simulink model "M10B39_V2"  (R2025a)
settings: Solver=ode23tb  StartTime=0.0  StopTime=1000  FixedStep=0.001  RelTol=1e-3  EnableMultiTasking=on
InitFcn:
  | clear;
  | initAll_V2;
  | %set_param('M10B39/Python2Sim','value','zeros(1,16)');
values from neighbouring files (symbols this model uses):
  acom = 100    [initAll.m]    (also in initAll_V2.m)
  bcom = 50    [initAll.m]    (also in initAll_V2.m)
  commun = 0*commun    [initAll.m]    (also in initAll_V2.m)
  DataDelay = 0.0*DataDelay    [initAll.m]    (also in initAll_V2.m)
  fB = 50    [initAll.m]    (also in initAll_V2.m)
  Geninit = Generator_init(opdata,SynMach_in_gidx)    [initAll.m]    (also in initAll_V2.m)
  lam = 100    [initAll.m]    (also in initAll_V2.m)
  loadnode = 31    [initAll_V2.m]
  loadsize = 16.2714    [initAll_V2.m]
  SgridB = 100    [initAll.m]    (also in initAll_V2.m)
  wB = 2*pi*fB    (= 314.159265359)    [initAll.m]    (also in initAll_V2.m)
undefined symbols (not defined in the file or in its folder): AVm0, c1, c2, c3, c4, c5, c6, cp_nom, ESinit, lambda_nom, P_wind_base, Pelec_base, Pnom, Windinit, YY_load
libraries: spsBistableLib x13, simulink_extras x5, powerlib_meascontrol x2, simulink x1
(part 2 of 11)

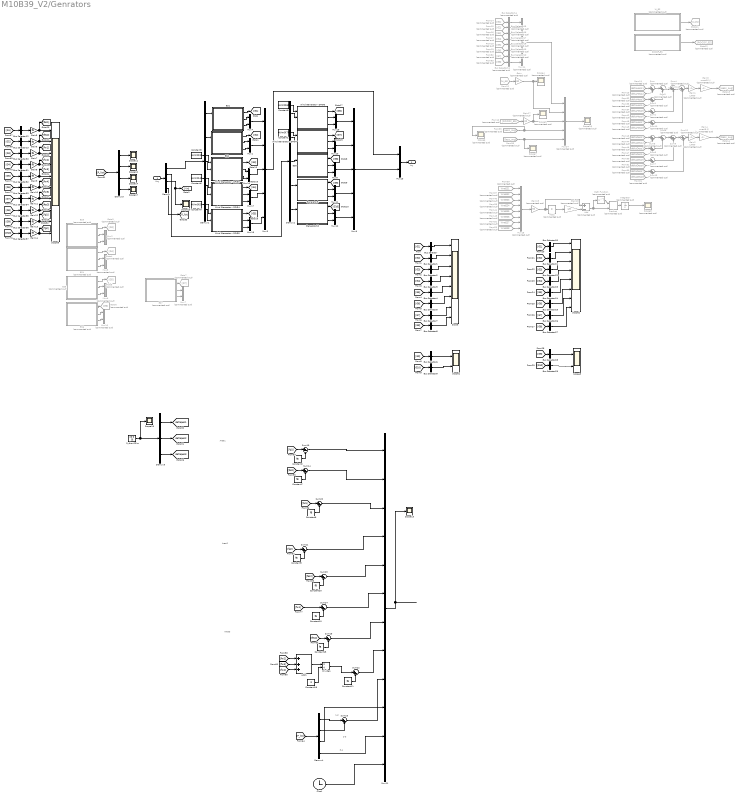
== system M10B39_V2/Genrators ==
  note: 3-1
  note: Area3
  note: 1-2
  note: 2-3
  note: Area2
  note: Area1
  Vxy : Inport
  Add : Sum  Commented=on  Inputs=+-
  Add1 : Sum  Inputs=+++
  Add2 : Sum  Commented=on  Inputs=+
  Bus Selector{,1..5,7..8,12..13,30..35} (16 alike) : BusSelector  OutputSignals=w
  Bus Selector{10..11,14..19} (8 alike) : BusSelector  Commented=on  OutputSignals=Pe
  Bus Selector{20..29} (10 alike) : BusSelector  OutputSignals=Pe
  Bus Selector{6,9,36..37} (4 alike) : BusSelector  OutputSignals=f
  Clock : Clock
  Constant1 : Constant  Value=AVm0(7)
  Constant{2,7..11,15,20} (8 alike) : Constant  Value=fB
  Constant18 : Constant  Value=3
  Constant3 : Constant  Value=AVm0(3)
  Constant4 : Constant  Value=AVm0(5)
  Constant5 : Constant  Value=AVm0(6)
  Constant6 : Constant  Value=AVm0(4)
  Demux : Demux  Outputs=[10 10 29 4]
      settings: DisplayOption=none
  Demux1 : Demux  Outputs=5
      settings: DisplayOption=none
  Demux2 : Demux  Outputs=5
      settings: DisplayOption=none
  Demux3 : Demux
  Demux4 : Demux
  Demux5 : Demux  Outputs=3
  Divide1 : Product  Inputs=*/
  ES1 : Subsystem  mask{SvscB=ESinit.SvscBi(1), SgridB=SgridB, Kppll_VSC=ESinit.Kppll(1), Kipll_VSC=ESinit.Kipll(1), Dels_hvdc=ESinit.Dels_hvdc(1), Lpr=ESinit.Lpr(1), Rpr=ESinit.Rpr(1), wB=wB, Is_xA_0=ESinit.Isx0(1), Is_yA_0=ESinit.Isy0(1), KpP_VSC_A=ESinit.KpP(1), KiP_VSC_A=ESinit.KiP(1), KpId_VSC_A=ESinit.KpId(1), KiId_VSC_A=ESinit.KiId(1), KpQ_VSC_A=ESinit.KpQ(1), KiQ_VSC_A=ESinit.KiQ(1), KpIq_VSC_A=ESinit.KpIq(1), KiIq_VSC_A=ESinit.KiIq(1), Md_A_0=ESinit.Md0(1), Mq_A_0=ESinit.Mq0(1), Nd_A_0=ESinit.Nd0(1), Nq_A_0=ESinit.Nq0(1), KIR=ESinit.Kir(1), Kdroop=ESinit.Kdroop(1), Kdistributed=ESinit.Kdistributed(1), Kdistributed_d=ESinit.Kdistributed_d(1), Kpac_VSC_A=ESinit.Kpac(1), Kiac_VSC_A=ESinit.Kiac(1), P0=ESinit.P0(1), Q0=ESinit.Q0(1), usd0=ESinit.Usd0(1)}
      mask prompts: Kppll_VSC "Kppll"; Kipll_VSC "Kipll"; KpP_VSC_A "KpP"; KiP_VSC_A "KiP"; KpId_VSC_A "KpId"; KiId_VSC_A "KiId"; KpQ_VSC_A "KpQ"; KiQ_VSC_A "KiQ"; KpIq_VSC_A "KpIq"; KiIq_VSC_A "KiIq"; Kpac_VSC_A "Kpac"; Kiac_VSC_A "Kiac"
      mask DialogControl Container48 Prompt: Base value
      mask DialogControl Container7 Prompt: PLL
      mask DialogControl Container5 Prompt: Control parameter
      mask DialogControl Container8 Prompt: inital value
      mask DialogControl Container9 Prompt: AC side
      mask DialogControl Container10 Prompt: Parameter
      mask DialogControl Container11 Prompt: Initial value
      mask DialogControl Container18 Prompt: Control parameter
      mask DialogControl Container19 Prompt: d_axis_control parameter
      mask DialogControl Container23 Prompt: d_axis_control=1
      mask DialogControl Container26 Prompt: inner current control
      mask DialogControl Container21 Prompt: q_axis_control parameter
      mask DialogControl Container29 Prompt: q_axis_control=1
      mask DialogControl Container31 Prompt: inner current control
      mask DialogControl Container22 Prompt: inital value
      mask DialogControl Container35 Prompt: outer controller
      mask DialogControl Container36 Prompt: inner control
      mask DialogControl Container27 Prompt: Inertia control
      mask DialogControl Container28 Prompt: droop control
      mask DialogControl Container300 Prompt: distributed control
      mask DialogControl Container301 Prompt: Droop distributed control
      mask DialogControl Container40 Prompt: usdq_control
      mask DialogControl Container41 Prompt: PQinitial
      mask DialogControl Container42 Prompt: usd0initial
  ES2 : Subsystem  mask{SvscB=ESinit.SvscBi(2), SgridB=SgridB, Kppll_VSC=ESinit.Kppll(2), Kipll_VSC=ESinit.Kipll(2), Dels_hvdc=ESinit.Dels_hvdc(2), Lpr=ESinit.Lpr(2), Rpr=ESinit.Rpr(2), wB=wB, Is_xA_0=ESinit.Isx0(2), Is_yA_0=ESinit.Isy0(2), KpP_VSC_A=ESinit.KpP(2), KiP_VSC_A=ESinit.KiP(2), KpId_VSC_A=ESinit.KpId(2), KiId_VSC_A=ESinit.KiId(2), KpQ_VSC_A=ESinit.KpQ(2), KiQ_VSC_A=ESinit.KiQ(2), KpIq_VSC_A=ESinit.KpIq(2), KiIq_VSC_A=ESinit.KiIq(2), Md_A_0=ESinit.Md0(2), Mq_A_0=ESinit.Mq0(2), Nd_A_0=ESinit.Nd0(2), Nq_A_0=ESinit.Nq0(2), KIR=ESinit.Kir(2), Kdroop=ESinit.Kdroop(2), Kdistributed=ESinit.Kdistributed(2), Kdistributed_d=ESinit.Kdistributed_d(2), Kpac_VSC_A=ESinit.Kpac(2), Kiac_VSC_A=ESinit.Kiac(2), P0=ESinit.P0(2), Q0=ESinit.Q0(2), usd0=ESinit.Usd0(2)}
      mask prompts: Kppll_VSC "Kppll"; Kipll_VSC "Kipll"; KpP_VSC_A "KpP"; KiP_VSC_A "KiP"; KpId_VSC_A "KpId"; KiId_VSC_A "KiId"; KpQ_VSC_A "KpQ"; KiQ_VSC_A "KiQ"; KpIq_VSC_A "KpIq"; KiIq_VSC_A "KiIq"; Kpac_VSC_A "Kpac"; Kiac_VSC_A "Kiac"
      mask DialogControl Container48 Prompt: Base value
      mask DialogControl Container7 Prompt: PLL
      mask DialogControl Container5 Prompt: Control parameter
      mask DialogControl Container8 Prompt: inital value
      mask DialogControl Container9 Prompt: AC side
      mask DialogControl Container10 Prompt: Parameter
      mask DialogControl Container11 Prompt: Initial value
      mask DialogControl Container18 Prompt: Control parameter
      mask DialogControl Container19 Prompt: d_axis_control parameter
      mask DialogControl Container23 Prompt: d_axis_control=1
      mask DialogControl Container26 Prompt: inner current control
      mask DialogControl Container21 Prompt: q_axis_control parameter
      mask DialogControl Container29 Prompt: q_axis_control=1
      mask DialogControl Container31 Prompt: inner current control
      mask DialogControl Container22 Prompt: inital value
      mask DialogControl Container35 Prompt: outer controller
      mask DialogControl Container36 Prompt: inner control
      mask DialogControl Container27 Prompt: Inertia control
      mask DialogControl Container28 Prompt: droop control
      mask DialogControl Container300 Prompt: distributed control
      mask DialogControl Container301 Prompt: Droop distributed control
      mask DialogControl Container40 Prompt: usdq_control
      mask DialogControl Container41 Prompt: PQinitial
      mask DialogControl Container42 Prompt: usd0initial
  ES3 : Subsystem  Commented=on  mask{SvscB=ESinit.SvscBi(3), SgridB=SgridB, Kppll_VSC=ESinit.Kppll(3), Kipll_VSC=ESinit.Kipll(3), Dels_hvdc=ESinit.Dels_hvdc(3), Lpr=ESinit.Lpr(3), Rpr=ESinit.Rpr(3), wB=wB, Is_xA_0=ESinit.Isx0(3), Is_yA_0=ESinit.Isy0(3), KpP_VSC_A=ESinit.KpP(3), KiP_VSC_A=ESinit.KiP(3), KpId_VSC_A=ESinit.KpId(3), KiId_VSC_A=ESinit.KiId(3), KpQ_VSC_A=ESinit.KpQ(3), KiQ_VSC_A=ESinit.KiQ(3), KpIq_VSC_A=ESinit.KpIq(3), KiIq_VSC_A=ESinit.KiIq(3), Md_A_0=ESinit.Md0(3), Mq_A_0=ESinit.Mq0(3), Nd_A_0=ESinit.Nd0(3), Nq_A_0=ESinit.Nq0(3), KIR=ESinit.Kir(3), Kdroop=ESinit.Kdroop(3), Kdistributed=ESinit.Kdistributed(3), Kdistributed_d=ESinit.Kdistributed_d(3), Kpac_VSC_A=ESinit.Kpac(3), Kiac_VSC_A=ESinit.Kiac(3), P0=ESinit.P0(3), Q0=ESinit.Q0(3), usd0=ESinit.Usd0(3)}
      mask prompts: Kppll_VSC "Kppll"; Kipll_VSC "Kipll"; KpP_VSC_A "KpP"; KiP_VSC_A "KiP"; KpId_VSC_A "KpId"; KiId_VSC_A "KiId"; KpQ_VSC_A "KpQ"; KiQ_VSC_A "KiQ"; KpIq_VSC_A "KpIq"; KiIq_VSC_A "KiIq"; Kpac_VSC_A "Kpac"; Kiac_VSC_A "Kiac"
      mask DialogControl Container48 Prompt: Base value
      mask DialogControl Container7 Prompt: PLL
      mask DialogControl Container5 Prompt: Control parameter
      mask DialogControl Container8 Prompt: inital value
      mask DialogControl Container9 Prompt: AC side
      mask DialogControl Container10 Prompt: Parameter
      mask DialogControl Container11 Prompt: Initial value
      mask DialogControl Container18 Prompt: Control parameter
      mask DialogControl Container19 Prompt: d_axis_control parameter
      mask DialogControl Container23 Prompt: d_axis_control=1
      mask DialogControl Container26 Prompt: inner current control
      mask DialogControl Container21 Prompt: q_axis_control parameter
      mask DialogControl Container29 Prompt: q_axis_control=1
      mask DialogControl Container31 Prompt: inner current control
      mask DialogControl Container22 Prompt: inital value
      mask DialogControl Container35 Prompt: outer controller
      mask DialogControl Container36 Prompt: inner control
      mask DialogControl Container27 Prompt: Inertia control
      mask DialogControl Container28 Prompt: droop control
      mask DialogControl Container300 Prompt: distributed control
      mask DialogControl Container301 Prompt: Droop distributed control
      mask DialogControl Container40 Prompt: usdq_control
      mask DialogControl Container41 Prompt: PQinitial
      mask DialogControl Container42 Prompt: usd0initial
  ES4 : Subsystem  Commented=on  mask{SvscB=ESinit.SvscBi(4), SgridB=SgridB, Kppll_VSC=ESinit.Kppll(4), Kipll_VSC=ESinit.Kipll(4), Dels_hvdc=ESinit.Dels_hvdc(4), Lpr=ESinit.Lpr(4), Rpr=ESinit.Rpr(4), wB=wB, Is_xA_0=ESinit.Isx0(4), Is_yA_0=ESinit.Isy0(4), KpP_VSC_A=ESinit.KpP(4), KiP_VSC_A=ESinit.KiP(4), KpId_VSC_A=ESinit.KpId(4), KiId_VSC_A=ESinit.KiId(4), KpQ_VSC_A=ESinit.KpQ(4), KiQ_VSC_A=ESinit.KiQ(4), KpIq_VSC_A=ESinit.KpIq(4), KiIq_VSC_A=ESinit.KiIq(4), Md_A_0=ESinit.Md0(4), Mq_A_0=ESinit.Mq0(4), Nd_A_0=ESinit.Nd0(4), Nq_A_0=ESinit.Nq0(4), KIR=ESinit.Kir(4), Kdroop=ESinit.Kdroop(4), Kdistributed=ESinit.Kdistributed(4), Kdistributed_d=ESinit.Kdistributed_d(4), Kpac_VSC_A=ESinit.Kpac(4), Kiac_VSC_A=ESinit.Kiac(4), P0=ESinit.P0(4), Q0=ESinit.Q0(4), usd0=ESinit.Usd0(4)}
      mask prompts: Kppll_VSC "Kppll"; Kipll_VSC "Kipll"; KpP_VSC_A "KpP"; KiP_VSC_A "KiP"; KpId_VSC_A "KpId"; KiId_VSC_A "KiId"; KpQ_VSC_A "KpQ"; KiQ_VSC_A "KiQ"; KpIq_VSC_A "KpIq"; KiIq_VSC_A "KiIq"; Kpac_VSC_A "Kpac"; Kiac_VSC_A "Kiac"
      mask DialogControl Container48 Prompt: Base value
      mask DialogControl Container7 Prompt: PLL
      mask DialogControl Container5 Prompt: Control parameter
      mask DialogControl Container8 Prompt: inital value
      mask DialogControl Container9 Prompt: AC side
      mask DialogControl Container10 Prompt: Parameter
      mask DialogControl Container11 Prompt: Initial value
      mask DialogControl Container18 Prompt: Control parameter
      mask DialogControl Container19 Prompt: d_axis_control parameter
      mask DialogControl Container23 Prompt: d_axis_control=1
      mask DialogControl Container26 Prompt: inner current control
      mask DialogControl Container21 Prompt: q_axis_control parameter
      mask DialogControl Container29 Prompt: q_axis_control=1
      mask DialogControl Container31 Prompt: inner current control
      mask DialogControl Container22 Prompt: inital value
      mask DialogControl Container35 Prompt: outer controller
      mask DialogControl Container36 Prompt: inner control
      mask DialogControl Container27 Prompt: Inertia control
      mask DialogControl Container28 Prompt: droop control
      mask DialogControl Container300 Prompt: distributed control
      mask DialogControl Container301 Prompt: Droop distributed control
      mask DialogControl Container40 Prompt: usdq_control
      mask DialogControl Container41 Prompt: PQinitial
      mask DialogControl Container42 Prompt: usd0initial
  ES5 : Subsystem  Commented=on  mask{SvscB=ESinit.SvscBi(5), SgridB=SgridB, Kppll_VSC=ESinit.Kppll(5), Kipll_VSC=ESinit.Kipll(5), Dels_hvdc=ESinit.Dels_hvdc(5), Lpr=ESinit.Lpr(5), Rpr=ESinit.Rpr(5), wB=wB, Is_xA_0=ESinit.Isx0(5), Is_yA_0=ESinit.Isy0(5), KpP_VSC_A=ESinit.KpP(5), KiP_VSC_A=ESinit.KiP(5), KpId_VSC_A=ESinit.KpId(5), KiId_VSC_A=ESinit.KiId(5), KpQ_VSC_A=ESinit.KpQ(5), KiQ_VSC_A=ESinit.KiQ(5), KpIq_VSC_A=ESinit.KpIq(5), KiIq_VSC_A=ESinit.KiIq(5), Md_A_0=ESinit.Md0(5), Mq_A_0=ESinit.Mq0(5), Nd_A_0=ESinit.Nd0(5), Nq_A_0=ESinit.Nq0(5), KIR=ESinit.Kir(5), Kdroop=ESinit.Kdroop(5), Kdistributed=ESinit.Kdistributed(5), Kdistributed_d=ESinit.Kdistributed_d(5), Kpac_VSC_A=ESinit.Kpac(5), Kiac_VSC_A=ESinit.Kiac(5), P0=ESinit.P0(5), Q0=ESinit.Q0(5), usd0=ESinit.Usd0(5)}
      mask prompts: Kppll_VSC "Kppll"; Kipll_VSC "Kipll"; KpP_VSC_A "KpP"; KiP_VSC_A "KiP"; KpId_VSC_A "KpId"; KiId_VSC_A "KiId"; KpQ_VSC_A "KpQ"; KiQ_VSC_A "KiQ"; KpIq_VSC_A "KpIq"; KiIq_VSC_A "KiIq"; Kpac_VSC_A "Kpac"; Kiac_VSC_A "Kiac"
      mask DialogControl Container48 Prompt: Base value
      mask DialogControl Container7 Prompt: PLL
      mask DialogControl Container5 Prompt: Control parameter
      mask DialogControl Container8 Prompt: inital value
      mask DialogControl Container9 Prompt: AC side
      mask DialogControl Container10 Prompt: Parameter
      mask DialogControl Container11 Prompt: Initial value
      mask DialogControl Container18 Prompt: Control parameter
      mask DialogControl Container19 Prompt: d_axis_control parameter
      mask DialogControl Container23 Prompt: d_axis_control=1
      mask DialogControl Container26 Prompt: inner current control
      mask DialogControl Container21 Prompt: q_axis_control parameter
      mask DialogControl Container29 Prompt: q_axis_control=1
      mask DialogControl Container31 Prompt: inner current control
      mask DialogControl Container22 Prompt: inital value
      mask DialogControl Container35 Prompt: outer controller
      mask DialogControl Container36 Prompt: inner control
      mask DialogControl Container27 Prompt: Inertia control
      mask DialogControl Container28 Prompt: droop control
      mask DialogControl Container300 Prompt: distributed control
      mask DialogControl Container301 Prompt: Droop distributed control
      mask DialogControl Container40 Prompt: usdq_control
      mask DialogControl Container41 Prompt: PQinitial
      mask DialogControl Container42 Prompt: usd0initial
  ES6 : Subsystem  Commented=on  mask{SvscB=ESinit.SvscBi(6), SgridB=SgridB, Kppll_VSC=ESinit.Kppll(6), Kipll_VSC=ESinit.Kipll(6), Dels_hvdc=ESinit.Dels_hvdc(6), Lpr=ESinit.Lpr(6), Rpr=ESinit.Rpr(6), wB=wB, Is_xA_0=ESinit.Isx0(6), Is_yA_0=ESinit.Isy0(6), KpP_VSC_A=ESinit.KpP(6), KiP_VSC_A=ESinit.KiP(6), KpId_VSC_A=ESinit.KpId(6), KiId_VSC_A=ESinit.KiId(6), KpQ_VSC_A=ESinit.KpQ(6), KiQ_VSC_A=ESinit.KiQ(6), KpIq_VSC_A=ESinit.KpIq(6), KiIq_VSC_A=ESinit.KiIq(6), Md_A_0=ESinit.Md0(6), Mq_A_0=ESinit.Mq0(6), Nd_A_0=ESinit.Nd0(6), Nq_A_0=ESinit.Nq0(6), KIR=ESinit.Kir(6), Kdroop=ESinit.Kdroop(6), Kdistributed=ESinit.Kdistributed(6), Kdistributed_d=ESinit.Kdistributed_d(6), Kpac_VSC_A=ESinit.Kpac(6), Kiac_VSC_A=ESinit.Kiac(6), P0=ESinit.P0(6), Q0=ESinit.Q0(6), usd0=ESinit.Usd0(6)}
      mask prompts: Kppll_VSC "Kppll"; Kipll_VSC "Kipll"; KpP_VSC_A "KpP"; KiP_VSC_A "KiP"; KpId_VSC_A "KpId"; KiId_VSC_A "KiId"; KpQ_VSC_A "KpQ"; KiQ_VSC_A "KiQ"; KpIq_VSC_A "KpIq"; KiIq_VSC_A "KiIq"; Kpac_VSC_A "Kpac"; Kiac_VSC_A "Kiac"
      mask DialogControl Container48 Prompt: Base value
      mask DialogControl Container7 Prompt: PLL
      mask DialogControl Container5 Prompt: Control parameter
      mask DialogControl Container8 Prompt: inital value
      mask DialogControl Container9 Prompt: AC side
      mask DialogControl Container10 Prompt: Parameter
      mask DialogControl Container11 Prompt: Initial value
      mask DialogControl Container18 Prompt: Control parameter
      mask DialogControl Container19 Prompt: d_axis_control parameter
      mask DialogControl Container23 Prompt: d_axis_control=1
      mask DialogControl Container26 Prompt: inner current control
      mask DialogControl Container21 Prompt: q_axis_control parameter
      mask DialogControl Container29 Prompt: q_axis_control=1
      mask DialogControl Container31 Prompt: inner current control
      mask DialogControl Container22 Prompt: inital value
      mask DialogControl Container35 Prompt: outer controller
      mask DialogControl Container36 Prompt: inner control
      mask DialogControl Container27 Prompt: Inertia control
      mask DialogControl Container28 Prompt: droop control
      mask DialogControl Container300 Prompt: distributed control
      mask DialogControl Container301 Prompt: Droop distributed control
      mask DialogControl Container40 Prompt: usdq_control
      mask DialogControl Container41 Prompt: PQinitial
      mask DialogControl Container42 Prompt: usd0initial
  ES7 : Subsystem  Commented=on  mask{SvscB=ESinit.SvscBi(7), SgridB=SgridB, Kppll_VSC=ESinit.Kppll(7), Kipll_VSC=ESinit.Kipll(7), Dels_hvdc=ESinit.Dels_hvdc(7), Lpr=ESinit.Lpr(7), Rpr=ESinit.Rpr(7), wB=wB, Is_xA_0=ESinit.Isx0(7), Is_yA_0=ESinit.Isy0(7), KpP_VSC_A=ESinit.KpP(7), KiP_VSC_A=ESinit.KiP(7), KpId_VSC_A=ESinit.KpId(7), KiId_VSC_A=ESinit.KiId(7), KpQ_VSC_A=ESinit.KpQ(7), KiQ_VSC_A=ESinit.KiQ(7), KpIq_VSC_A=ESinit.KpIq(7), KiIq_VSC_A=ESinit.KiIq(7), Md_A_0=ESinit.Md0(7), Mq_A_0=ESinit.Mq0(7), Nd_A_0=ESinit.Nd0(7), Nq_A_0=ESinit.Nq0(7), KIR=ESinit.Kir(7), Kdroop=ESinit.Kdroop(7), Kdistributed=ESinit.Kdistributed(7), Kdistributed_d=ESinit.Kdistributed_d(7), Kpac_VSC_A=ESinit.Kpac(7), Kiac_VSC_A=ESinit.Kiac(7), P0=ESinit.P0(7), Q0=ESinit.Q0(7), usd0=ESinit.Usd0(7)}
      mask prompts: Kppll_VSC "Kppll"; Kipll_VSC "Kipll"; KpP_VSC_A "KpP"; KiP_VSC_A "KiP"; KpId_VSC_A "KpId"; KiId_VSC_A "KiId"; KpQ_VSC_A "KpQ"; KiQ_VSC_A "KiQ"; KpIq_VSC_A "KpIq"; KiIq_VSC_A "KiIq"; Kpac_VSC_A "Kpac"; Kiac_VSC_A "Kiac"
      mask DialogControl Container48 Prompt: Base value
      mask DialogControl Container7 Prompt: PLL
      mask DialogControl Container5 Prompt: Control parameter
      mask DialogControl Container8 Prompt: inital value
      mask DialogControl Container9 Prompt: AC side
      mask DialogControl Container10 Prompt: Parameter
      mask DialogControl Container11 Prompt: Initial value
      mask DialogControl Container18 Prompt: Control parameter
      mask DialogControl Container19 Prompt: d_axis_control parameter
      mask DialogControl Container23 Prompt: d_axis_control=1
      mask DialogControl Container26 Prompt: inner current control
      mask DialogControl Container21 Prompt: q_axis_control parameter
      mask DialogControl Container29 Prompt: q_axis_control=1
      mask DialogControl Container31 Prompt: inner current control
      mask DialogControl Container22 Prompt: inital value
      mask DialogControl Container35 Prompt: outer controller
      mask DialogControl Container36 Prompt: inner control
      mask DialogControl Container27 Prompt: Inertia control
      mask DialogControl Container28 Prompt: droop control
      mask DialogControl Container300 Prompt: distributed control
      mask DialogControl Container301 Prompt: Droop distributed control
      mask DialogControl Container40 Prompt: usdq_control
      mask DialogControl Container41 Prompt: PQinitial
      mask DialogControl Container42 Prompt: usd0initial
  ES8 : Subsystem  mask{SvscB=ESinit.SvscBi(8), SgridB=SgridB, Kppll_VSC=ESinit.Kppll(8), Kipll_VSC=ESinit.Kipll(8), Dels_hvdc=ESinit.Dels_hvdc(8), Lpr=ESinit.Lpr(8), Rpr=ESinit.Rpr(8), wB=wB, Is_xA_0=ESinit.Isx0(8), Is_yA_0=ESinit.Isy0(8), KpP_VSC_A=ESinit.KpP(8), KiP_VSC_A=ESinit.KiP(8), KpId_VSC_A=ESinit.KpId(8), KiId_VSC_A=ESinit.KiId(8), KpQ_VSC_A=ESinit.KpQ(8), KiQ_VSC_A=ESinit.KiQ(8), KpIq_VSC_A=ESinit.KpIq(8), KiIq_VSC_A=ESinit.KiIq(8), Md_A_0=ESinit.Md0(8), Mq_A_0=ESinit.Mq0(8), Nd_A_0=ESinit.Nd0(8), Nq_A_0=ESinit.Nq0(8), KIR=ESinit.Kir(8), Kdroop=ESinit.Kdroop(8), Kdistributed=ESinit.Kdistributed(8), Kdistributed_d=ESinit.Kdistributed_d(8), Kpac_VSC_A=ESinit.Kpac(8), Kiac_VSC_A=ESinit.Kiac(8), P0=ESinit.P0(8), Q0=ESinit.Q0(8), usd0=ESinit.Usd0(8)}
      mask prompts: Kppll_VSC "Kppll"; Kipll_VSC "Kipll"; KpP_VSC_A "KpP"; KiP_VSC_A "KiP"; KpId_VSC_A "KpId"; KiId_VSC_A "KiId"; KpQ_VSC_A "KpQ"; KiQ_VSC_A "KiQ"; KpIq_VSC_A "KpIq"; KiIq_VSC_A "KiIq"; Kpac_VSC_A "Kpac"; Kiac_VSC_A "Kiac"
      mask DialogControl Container48 Prompt: Base value
      mask DialogControl Container7 Prompt: PLL
      mask DialogControl Container5 Prompt: Control parameter
      mask DialogControl Container8 Prompt: inital value
      mask DialogControl Container9 Prompt: AC side
      mask DialogControl Container10 Prompt: Parameter
      mask DialogControl Container11 Prompt: Initial value
      mask DialogControl Container18 Prompt: Control parameter
      mask DialogControl Container19 Prompt: d_axis_control parameter
      mask DialogControl Container23 Prompt: d_axis_control=1
      mask DialogControl Container26 Prompt: inner current control
      mask DialogControl Container21 Prompt: q_axis_control parameter
      mask DialogControl Container29 Prompt: q_axis_control=1
      mask DialogControl Container31 Prompt: inner current control
      mask DialogControl Container22 Prompt: inital value
      mask DialogControl Container35 Prompt: outer controller
      mask DialogControl Container36 Prompt: inner control
      mask DialogControl Container27 Prompt: Inertia control
      mask DialogControl Container28 Prompt: droop control
      mask DialogControl Container300 Prompt: distributed control
      mask DialogControl Container301 Prompt: Droop distributed control
      mask DialogControl Container40 Prompt: usdq_control
      mask DialogControl Container41 Prompt: PQinitial
      mask DialogControl Container42 Prompt: usd0initial
  From10 : From  Commented=on  GotoTag=ROCOF_ES
  From11 : From  Commented=on  GotoTag=deltaHess1  TagVisibility=global
  From12 : From  Commented=on  GotoTag=W_ES
  From13 : From  Commented=on  GotoTag=deltaHess2  TagVisibility=global
  From14 : From  Commented=on  GotoTag=G1
  From15 : From  Commented=on  GotoTag=G2
  From16 : From  Commented=on  GotoTag=G3
  From17 : From  Commented=on  GotoTag=G4
  From18 : From  Commented=on  GotoTag=G5
  From19 : From  Commented=on  GotoTag=G6
  From30 : From  Commented=on  GotoTag=deltaDess5  TagVisibility=global
  From31 : From  Commented=on  GotoTag=deltaDess6  TagVisibility=global
  From32 : From  Commented=on  GotoTag=deltaHess3  TagVisibility=global
  From33 : From  Commented=on  GotoTag=deltaHess4  TagVisibility=global
  From34 : From  Commented=on  GotoTag=deltaHess5  TagVisibility=global
  From35 : From  Commented=on  GotoTag=Hess_avg
  From36 : From  Commented=on  GotoTag=Dess_avg
  From37 : From  Commented=on  GotoTag=WreES2  TagVisibility=global
  From38 : From  Commented=on  GotoTag=WreES4  TagVisibility=global
  From39 : From  Commented=on  GotoTag=WreES1  TagVisibility=global
  From40 : From  Commented=on  GotoTag=WreES3  TagVisibility=global
  From41 : From  Commented=on  GotoTag=WreES5  TagVisibility=global
  From42 : From  Commented=on  GotoTag=deltaHess6  TagVisibility=global
  From43 : From  Commented=on  GotoTag=deltaDess1  TagVisibility=global
  From44 : From  Commented=on  GotoTag=deltaDess2  TagVisibility=global
  From45 : From  Commented=on  GotoTag=WreES6  TagVisibility=global
  From46 : From  Commented=on  GotoTag=deltaDess3  TagVisibility=global
  From47 : From  Commented=on  GotoTag=deltaDess4  TagVisibility=global
  From48 : From  Commented=on  GotoTag=deltaHess7  TagVisibility=global
  From49 : From  Commented=on  GotoTag=deltaHess8  TagVisibility=global
  From50 : From  Commented=on  GotoTag=deltaDess7  TagVisibility=global
  From51 : From  Commented=on  GotoTag=deltaDess8  TagVisibility=global
  From52 : From  Commented=on  GotoTag=WreES7  TagVisibility=global
  From53 : From  Commented=on  GotoTag=WreES8  TagVisibility=global
  From82 : From  Commented=on  GotoTag=G7
  From83 : From  Commented=on  GotoTag=G8
  Gain : Gain  Commented=on  Gain=80
  Gain1 : Gain  Commented=on  Gain=1/800
  Gain{5..14} (10 alike) : Gain  Gain=fB
  Gain17 : Gain  Commented=on  Gain=20
  Gain18 : Gain  Commented=on  Gain=1/8
  Gain19 : Gain  Commented=on  Gain=50
  Gain2 : Gain  Commented=on  Gain=1/800
  Gain3 : Gain  Commented=on  Gain=ones(8,1)
  Gain4 : Gain  Commented=on  Gain=ones(8,1)
  Generator10 : Subsystem  mask{wB=wB, SgenB=Geninit.SgenB(10), SgridB=SgridB, Xq=Geninit.Xq(10), Xq1=Geninit.Xq1(10), Xq11=Geninit.Xq11(10), Tq0=Geninit.Tq0(10), Tq10=Geninit.Tq10(10), Eq10=Geninit.Eq1(10), Eq110=Geninit.Eq11(10), Xd=Geninit.Xd(10), Xd1=Geninit.Xd1(10), Xd11=Geninit.Xd11(10), Td0=Geninit.Td0(10), Td10=Geninit.Td10(10), Ed10=Geninit.Ed1(10), Ed110=Geninit.Ed11(10), H=Geninit.Tj(10), D=Geninit.D(10), delta0=Geninit.Delta(10), w0=1, Pm0=Geninit.Pm0(10), Ka=Geninit.Ka(10), Tb=Geninit.Tb(10), Tc=Geninit.Tc(10), Efmax=Geninit.Efmax(10), Efmin=Geninit.Efmin(10), Vref=Geninit.Vref(10), Ef10=Geninit.Vf1(10), S_PSS=Geninit.EnablePSS(10), Kpss=Geninit.kpss(10), Tw_P=Geninit.Tw_P(10), T1_P=Geninit.T1_P(10), T2_P=Geninit.T2_P(10), T3_P=Geninit.T3_P(10), T4_P=Geninit.T4_P(10), Upmax=Geninit.Upmax(10), Upmin=Geninit.Upmin(10), S_Gov=Geninit.Enablegov(10), a_G=Geninit.a_G(10), b_G=Geninit.b_G(10), Tg_G=Geninit.Tg_G(10), dPmax=Geninit.dPmax(10), dPmin=Geninit.dPmin(10)}
      mask prompts: S_PSS "Enable PSS"; Tw_P "Tw"; T1_P "T1"; T2_P "T2"; T3_P "T3"; T4_P "T4"; S_Gov "Enable Governor"; a_G "a"; b_G "b"; Tg_G "Tg"
      mask help: This is a six-order synchronous generator with exciter system, governor and PSS.
      mask DialogControl Container6 Prompt: Machine parameter
      mask DialogControl Container3 Prompt: q axis parameter
      mask DialogControl ParameterGroupVar Prompt: d axis parameter
      mask DialogControl Container4 Prompt: machine parameter
      mask DialogControl Container12 Prompt: Excitation System parameter
      mask DialogControl Container20 Prompt: parameter
      mask DialogControl Container21 Prompt: inital value
      mask DialogControl Container10 Prompt: PSS parameter
      mask DialogControl Container13 Prompt: Governor parameter
  Generator9 : Subsystem  mask{wB=wB, SgenB=Geninit.SgenB(9), SgridB=SgridB, Xq=Geninit.Xq(9), Xq1=Geninit.Xq1(9), Xq11=Geninit.Xq11(9), Tq0=Geninit.Tq0(9), Tq10=Geninit.Tq10(9), Eq10=Geninit.Eq1(9), Eq110=Geninit.Eq11(9), Xd=Geninit.Xd(9), Xd1=Geninit.Xd1(9), Xd11=Geninit.Xd11(9), Td0=Geninit.Td0(9), Td10=Geninit.Td10(9), Ed10=Geninit.Ed1(9), Ed110=Geninit.Ed11(9), H=Geninit.Tj(9), D=Geninit.D(9), delta0=Geninit.Delta(9), w0=1, Pm0=Geninit.Pm0(9), Ka=Geninit.Ka(9), Tb=Geninit.Tb(9), Tc=Geninit.Tc(9), Efmax=Geninit.Efmax(9), Efmin=Geninit.Efmin(9), Vref=Geninit.Vref(9), Ef10=Geninit.Vf1(9), S_PSS=Geninit.EnablePSS(9), Kpss=Geninit.kpss(9), Tw_P=Geninit.Tw_P(9), T1_P=Geninit.T1_P(9), T2_P=Geninit.T2_P(9), T3_P=Geninit.T3_P(9), T4_P=Geninit.T4_P(9), Upmax=Geninit.Upmax(9), Upmin=Geninit.Upmin(9), S_Gov=Geninit.Enablegov(9), a_G=Geninit.a_G(9), b_G=Geninit.b_G(9), Tg_G=Geninit.Tg_G(9), dPmax=Geninit.dPmax(9), dPmin=Geninit.dPmin(9)}
      mask prompts: S_PSS "Enable PSS"; Tw_P "Tw"; T1_P "T1"; T2_P "T2"; T3_P "T3"; T4_P "T4"; S_Gov "Enable Governor"; a_G "a"; b_G "b"; Tg_G "Tg"
      mask help: This is a six-order synchronous generator with exciter system, governor and PSS.
      mask DialogControl Container6 Prompt: Machine parameter
      mask DialogControl Container3 Prompt: q axis parameter
      mask DialogControl ParameterGroupVar Prompt: d axis parameter
      mask DialogControl Container4 Prompt: machine parameter
      mask DialogControl Container12 Prompt: Excitation System parameter
      mask DialogControl Container20 Prompt: parameter
      mask DialogControl Container21 Prompt: inital value
      mask DialogControl Container10 Prompt: PSS parameter
      mask DialogControl Container13 Prompt: Governor parameter
  Goto11 : Goto  Commented=on  GotoTag=W_ES
  Goto12 : Goto  Commented=on  GotoTag=ROCOF_ES
  Goto13 : Goto  Commented=on  GotoTag=Hess_avg
  Goto14 : Goto  Commented=on  GotoTag=Dess_avg
  Goto3 : Goto  Commented=on  GotoTag=G3
  Goto4 : Goto  Commented=on  GotoTag=G4
  Goto5 : Goto  Commented=on  GotoTag=G5
  Goto6 : Goto  Commented=on  GotoTag=G6
  Goto7 : Goto  Commented=on  GotoTag=G7
  Integrator : Integrator  Commented=on
  Math Function : Math  Commented=on  Operator=transpose
  Mux{1,4,8,11..13,16..20} (11 alike) : Mux  Inputs=2
  Mux{2,5..7,10} (5 alike) : Mux  Commented=on  Inputs=2
  Mux14 : Mux  Commented=on  Inputs=8
  Mux15 : Mux  Commented=on  Inputs=8
  Mux21 : Mux  Inputs=12
  Mux24 : Mux  Commented=on  Inputs=5
  Mux3 : Mux  Inputs=5
  Mux9 : Mux  Inputs=5
  Product : Product  Commented=on  Multiplication=Matrix(*)
  Python2Sim : Constant  Value=[0 0 0]
  ROCOF_ES : Subsystem  Commented=on
  Scope : Scope  NumInputPorts=8
      settings: ActiveDisplayYMinimum=0.98800694276558265  ActiveDisplayYMaximum=1.0024602359301829
  Scope1 : Scope  NumInputPorts=2
      settings: ActiveDisplayYMinimum=0.999922338749743  ActiveDisplayYMaximum=1.0005500939980669
  Scope{10..15,17} (7 alike) : Scope
      Scope10 settings: ActiveDisplayYMinimum=0.98473  ActiveDisplayYMaximum=1.07242  DataLoggingVariableName=ScopeData4
      Scope11 settings: ActiveDisplayYMinimum=-0.27398046174881396  ActiveDisplayYMaximum=1.3463574821887458  DataLoggingVariableName=ScopeData24
      Scope12 settings: ActiveDisplayYMinimum=-0.18188603281064061  ActiveDisplayYMaximum=0.25432052788139309  DataLoggingVariableName=ScopeData26
      Scope13 settings: ActiveDisplayYMinimum=-20.35289  ActiveDisplayYMaximum=182.95724  DataLoggingVariableName=ScopeData21
      Scope14 settings: ActiveDisplayYMinimum=-1.1754062179527387  ActiveDisplayYMaximum=0.39017552592908222  DataLoggingVariableName=ScopeData27
      Scope15 settings: ActiveDisplayYMinimum=-1  ActiveDisplayYMaximum=1  DataLoggingVariableName=ScopeData20
      Scope17 settings: ActiveDisplayYMinimum=-0.84865036706656172  ActiveDisplayYMaximum=1.5666769677631582  DataLoggingVariableName=ScopeData19
  Scope{4..8,16} (6 alike) : Scope  Commented=on
      Scope16 settings: ActiveDisplayYMinimum=-0.65989  ActiveDisplayYMaximum=0.16966  DataLoggingVariableName=ScopeData3
      Scope4 settings: ActiveDisplayYMinimum=-12.70415  ActiveDisplayYMaximum=6.31422  DataLoggingVariableName=ScopeData2
      Scope5 settings: ActiveDisplayYMinimum=-8.85266  ActiveDisplayYMaximum=5.76211  DataLoggingVariableName=ScopeData4
      Scope6 settings: ActiveDisplayYMinimum=-0.04265  ActiveDisplayYMaximum=0.38387  DataLoggingVariableName=ScopeData5
      Scope7 settings: ActiveDisplayYMinimum=-1  ActiveDisplayYMaximum=1  DataLoggingVariableName=ScopeData6
      Scope8 settings: ActiveDisplayYMinimum=-6E-10  ActiveDisplayYMaximum=5.2E-9
  Scope2 : Scope  NumInputPorts=8
      settings: ActiveDisplayYMinimum=-0.36304883163896517  ActiveDisplayYMaximum=0.60273095924554043  DataLoggingVariableName=ScopeData3
  Scope3 : Scope  NumInputPorts=2
      settings: ActiveDisplayYMinimum=6.1743661088987478  ActiveDisplayYMaximum=30.854324881451046  DataLoggingVariableName=ScopeData2
  Scope9 : Scope  NumInputPorts=10
      settings: ActiveDisplayYMinimum=49.83673884010885  ActiveDisplayYMaximum=50.044024898477971  DataLoggingVariableName=ScopeData18
  Sum{,1..13} (14 alike) : Sum  Commented=on  Inputs=|++
  Sum{14..15,19..24} (8 alike) : Sum  Inputs=|+-
  Sum16 : Sum  Inputs=|++
  W_ES : Subsystem  Commented=on
  Wind Generator - DFIG3 : Subsystem  mask{NN=Windinit.NN(3), SwgBi=Windinit.SwgBi(3), SmecBi=100, SgridB=SgridB, Atheta=Windinit.Atheta(3), Kppll=Windinit.Kppll_wind(3), Kipll=Windinit.Kipll_wind(3), pitch=[500 45 2], Srotors=1.3, H=Windinit.H(3), Wr0=Windinit.Wr0(3), Xa=Windinit.Xa(3), Xa1=Windinit.Xa1(3), Lm=Windinit.Lm(3), Lr=Windinit.Lr(3), Rs=Windinit.Rs(3), Ls=Windinit.Ls(3), Ta0=Windinit.Ta0(3), NPf=Windinit.NPf(3), Za=Windinit.Za{3}, Ex0=Windinit.Ex_ref(3), Ey0=Windinit.Ey_ref(3), wB=wB, KpP_rw=Windinit.KpP_rw(3), KiP_rw=Windinit.KiP_rw(3), KpId_rw=Windinit.KpId_rw(3), KiId_rw=Windinit.KiId_rw(3), KpQ_rw=Windinit.KpQ_rw(3), KiQ_rw=Windinit.KiQ_rw(3), KpIq_rw=Windinit.KpIq_rw(3), KiIq_rw=Windinit.KiIq_rw(3), Ird_ref=Windinit.Ird_ref(3), Irq_ref=Windinit.Irq_ref(3), Qs0=Windinit.Qs0(3), KpDC_gw=Windinit.KpDC_gw(3), KiDC_gw=Windinit.KiDC_gw(3), KpId_gw=Windinit.KpId_gw(3), KiId_gw=Windinit.KiId_gw(3), KpIq_gw=Windinit.KpIq_gw(3), KiIq_gw=Windinit.KiIq_gw(2), Vdc_w=Windinit.Vdc_w(3), Icd_ref=Windinit.Icd_ref(3), Icq_ref=Windinit.Icq_ref(3), Vcd_ref=Windinit.Vcd_ref(3), Vcq_ref=Windinit.Vcq_ref(3), Lg=Windinit.Lg(3), Rg=Windinit.Rg(3), Icx0=Windinit.Icx0(3), Icy0=Windinit.Icy0(3), C_w=Windinit.C_w(3), Vdc0=Windinit.Vdc0(3)}
      mask prompts: pitch "pitch_gain，pitch_max，pitch_rate"; Srotors "Start Rotor Speed"; Ex0 "Ex"; Ey0 "Ey"
      mask init:
      | pitch_gain=pitch(1);
      | pitch_max=pitch(2);
      | pitch_rate=pitch(3);
      | 
      | %该风机模型的基准容量
      | 
      | SwgeqB=SwgBi.*NN;
      mask DialogControl Container4 Prompt: PLL/Wind turbine
      mask DialogControl Container31 Prompt: Base value
      mask DialogControl Container23 Prompt: PLL
      mask DialogControl Container6 Prompt: inital value
      mask DialogControl Container5 Prompt: PI parameter
      mask DialogControl Container24 Prompt: Wind turbine
      mask DialogControl Container25 Prompt: pitch control
      mask DialogControl Container7 Prompt: Machine parameter
      mask DialogControl Container8 Prompt: Rotor
      mask DialogControl Container9 Prompt: Machine
      mask DialogControl Container10 Prompt: parameter
      mask DialogControl Container11 Prompt: inital value
      mask DialogControl Container12 Prompt: Rotor side control
      mask DialogControl Container13 Prompt: Control parameter
      mask DialogControl Container14 Prompt: Initial value
      mask DialogControl Container15 Prompt: reactive power
      mask DialogControl Container16 Prompt: Grid side control
      mask DialogControl Container17 Prompt: parameter
      mask DialogControl Container18 Prompt: reference
      mask DialogControl Container19 Prompt: inital value
      mask DialogControl Container20 Prompt: converter function
      mask DialogControl Container21 Prompt: inital value
      mask DialogControl Container22 Prompt: DC function
  Wind Generator - DFIG4 : Subsystem  mask{NN=Windinit.NN(4), SwgBi=Windinit.SwgBi(4), SmecBi=100, SgridB=SgridB, Atheta=Windinit.Atheta(4), Kppll=Windinit.Kppll_wind(4), Kipll=Windinit.Kipll_wind(4), pitch=[500 45 2], Srotors=1.3, H=Windinit.H(4), Wr0=Windinit.Wr0(4), Xa=Windinit.Xa(4), Xa1=Windinit.Xa1(4), Lm=Windinit.Lm(4), Lr=Windinit.Lr(4), Rs=Windinit.Rs(4), Ls=Windinit.Ls(4), Ta0=Windinit.Ta0(4), NPf=Windinit.NPf(4), Za=Windinit.Za{4}, Ex0=Windinit.Ex_ref(4), Ey0=Windinit.Ey_ref(4), wB=wB, KpP_rw=Windinit.KpP_rw(4), KiP_rw=Windinit.KiP_rw(4), KpId_rw=Windinit.KpId_rw(4), KiId_rw=Windinit.KiId_rw(4), KpQ_rw=Windinit.KpQ_rw(4), KiQ_rw=Windinit.KiQ_rw(4), KpIq_rw=Windinit.KpIq_rw(4), KiIq_rw=Windinit.KiIq_rw(4), Ird_ref=Windinit.Ird_ref(4), Irq_ref=Windinit.Irq_ref(4), Qs0=Windinit.Qs0(4), KpDC_gw=Windinit.KpDC_gw(4), KiDC_gw=Windinit.KiDC_gw(4), KpId_gw=Windinit.KpId_gw(4), KiId_gw=Windinit.KiId_gw(4), KpIq_gw=Windinit.KpIq_gw(4), KiIq_gw=Windinit.KiIq_gw(4), Vdc_w=Windinit.Vdc_w(4), Icd_ref=Windinit.Icd_ref(4), Icq_ref=Windinit.Icq_ref(4), Vcd_ref=Windinit.Vcd_ref(4), Vcq_ref=Windinit.Vcq_ref(4), Lg=Windinit.Lg(4), Rg=Windinit.Rg(4), Icx0=Windinit.Icx0(4), Icy0=Windinit.Icy0(4), C_w=Windinit.C_w(4), Vdc0=Windinit.Vdc0(4)}
      mask prompts: pitch "pitch_gain，pitch_max，pitch_rate"; Srotors "Start Rotor Speed"; Ex0 "Ex"; Ey0 "Ey"
      mask init:
      | pitch_gain=pitch(1);
      | pitch_max=pitch(2);
      | pitch_rate=pitch(3);
      | 
      | %该风机模型的基准容量
      | 
      | SwgeqB=SwgBi.*NN;
      mask DialogControl Container4 Prompt: PLL/Wind turbine
      mask DialogControl Container31 Prompt: Base value
      mask DialogControl Container23 Prompt: PLL
      mask DialogControl Container6 Prompt: inital value
      mask DialogControl Container5 Prompt: PI parameter
      mask DialogControl Container24 Prompt: Wind turbine
      mask DialogControl Container25 Prompt: pitch control
      mask DialogControl Container7 Prompt: Machine parameter
      mask DialogControl Container8 Prompt: Rotor
      mask DialogControl Container9 Prompt: Machine
      mask DialogControl Container10 Prompt: parameter
      mask DialogControl Container11 Prompt: inital value
      mask DialogControl Container12 Prompt: Rotor side control
      mask DialogControl Container13 Prompt: Control parameter
      mask DialogControl Container14 Prompt: Initial value
      mask DialogControl Container15 Prompt: reactive power
      mask DialogControl Container16 Prompt: Grid side control
      mask DialogControl Container17 Prompt: parameter
      mask DialogControl Container18 Prompt: reference
      mask DialogControl Container19 Prompt: inital value
      mask DialogControl Container20 Prompt: converter function
      mask DialogControl Container21 Prompt: inital value
      mask DialogControl Container22 Prompt: DC function
  Wind Generator - DFIG5 : Subsystem  mask{NN=Windinit.NN(5), SwgBi=Windinit.SwgBi(5), SmecBi=100, SgridB=SgridB, Atheta=Windinit.Atheta(5), Kppll=Windinit.Kppll_wind(5), Kipll=Windinit.Kipll_wind(5), pitch=[500 45 2], Srotors=1.3, H=Windinit.H(5), Wr0=Windinit.Wr0(5), Xa=Windinit.Xa(5), Xa1=Windinit.Xa1(5), Lm=Windinit.Lm(5), Lr=Windinit.Lr(5), Rs=Windinit.Rs(5), Ls=Windinit.Ls(5), Ta0=Windinit.Ta0(5), NPf=Windinit.NPf(5), Za=Windinit.Za{5}, Ex0=Windinit.Ex_ref(5), Ey0=Windinit.Ey_ref(5), wB=wB, KpP_rw=Windinit.KpP_rw(5), KiP_rw=Windinit.KiP_rw(5), KpId_rw=Windinit.KpId_rw(5), KiId_rw=Windinit.KiId_rw(5), KpQ_rw=Windinit.KpQ_rw(5), KiQ_rw=Windinit.KiQ_rw(5), KpIq_rw=Windinit.KpIq_rw(5), KiIq_rw=Windinit.KiIq_rw(5), Ird_ref=Windinit.Ird_ref(5), Irq_ref=Windinit.Irq_ref(5), Qs0=Windinit.Qs0(5), KpDC_gw=Windinit.KpDC_gw(5), KiDC_gw=Windinit.KiDC_gw(5), KpId_gw=Windinit.KpId_gw(5), KiId_gw=Windinit.KiId_gw(5), KpIq_gw=Windinit.KpIq_gw(5), KiIq_gw=Windinit.KiIq_gw(5), Vdc_w=Windinit.Vdc_w(5), Icd_ref=Windinit.Icd_ref(5), Icq_ref=Windinit.Icq_ref(5), Vcd_ref=Windinit.Vcd_ref(5), Vcq_ref=Windinit.Vcq_ref(5), Lg=Windinit.Lg(5), Rg=Windinit.Rg(5), Icx0=Windinit.Icx0(5), Icy0=Windinit.Icy0(5), C_w=Windinit.C_w(5), Vdc0=Windinit.Vdc0(5)}
      mask prompts: pitch "pitch_gain，pitch_max，pitch_rate"; Srotors "Start Rotor Speed"; Ex0 "Ex"; Ey0 "Ey"
      mask init:
      | pitch_gain=pitch(1);
      | pitch_max=pitch(2);
      | pitch_rate=pitch(3);
      | 
      | %该风机模型的基准容量
      | 
      | SwgeqB=SwgBi.*NN;
      mask DialogControl Container4 Prompt: PLL/Wind turbine
      mask DialogControl Container31 Prompt: Base value
      mask DialogControl Container23 Prompt: PLL
      mask DialogControl Container6 Prompt: inital value
      mask DialogControl Container5 Prompt: PI parameter
      mask DialogControl Container24 Prompt: Wind turbine
      mask DialogControl Container25 Prompt: pitch control
      mask DialogControl Container7 Prompt: Machine parameter
      mask DialogControl Container8 Prompt: Rotor
      mask DialogControl Container9 Prompt: Machine
      mask DialogControl Container10 Prompt: parameter
      mask DialogControl Container11 Prompt: inital value
      mask DialogControl Container12 Prompt: Rotor side control
      mask DialogControl Container13 Prompt: Control parameter
      mask DialogControl Container14 Prompt: Initial value
      mask DialogControl Container15 Prompt: reactive power
      mask DialogControl Container16 Prompt: Grid side control
      mask DialogControl Container17 Prompt: parameter
      mask DialogControl Container18 Prompt: reference
      mask DialogControl Container19 Prompt: inital value
      mask DialogControl Container20 Prompt: converter function
      mask DialogControl Container21 Prompt: inital value
      mask DialogControl Container22 Prompt: DC function
  Wind Generator - DFIG6 : Subsystem  mask{NN=Windinit.NN(6), SwgBi=Windinit.SwgBi(6), SmecBi=100, SgridB=SgridB, Atheta=Windinit.Atheta(6), Kppll=Windinit.Kppll_wind(6), Kipll=Windinit.Kipll_wind(6), pitch=[500 45 2], Srotors=1.3, H=Windinit.H(6), Wr0=Windinit.Wr0(6), Xa=Windinit.Xa(6), Xa1=Windinit.Xa1(6), Lm=Windinit.Lm(6), Lr=Windinit.Lr(6), Rs=Windinit.Rs(6), Ls=Windinit.Ls(6), Ta0=Windinit.Ta0(6), NPf=Windinit.NPf(6), Za=Windinit.Za{6}, Ex0=Windinit.Ex_ref(6), Ey0=Windinit.Ey_ref(6), wB=wB, KpP_rw=Windinit.KpP_rw(6), KiP_rw=Windinit.KiP_rw(6), KpId_rw=Windinit.KpId_rw(6), KiId_rw=Windinit.KiId_rw(6), KpQ_rw=Windinit.KpQ_rw(6), KiQ_rw=Windinit.KiQ_rw(6), KpIq_rw=Windinit.KpIq_rw(6), KiIq_rw=Windinit.KiIq_rw(6), Ird_ref=Windinit.Ird_ref(6), Irq_ref=Windinit.Irq_ref(6), Qs0=Windinit.Qs0(6), KpDC_gw=Windinit.KpDC_gw(6), KiDC_gw=Windinit.KiDC_gw(6), KpId_gw=Windinit.KpId_gw(6), KiId_gw=Windinit.KiId_gw(6), KpIq_gw=Windinit.KpIq_gw(6), KiIq_gw=Windinit.KiIq_gw(6), Vdc_w=Windinit.Vdc_w(6), Icd_ref=Windinit.Icd_ref(6), Icq_ref=Windinit.Icq_ref(6), Vcd_ref=Windinit.Vcd_ref(6), Vcq_ref=Windinit.Vcq_ref(6), Lg=Windinit.Lg(6), Rg=Windinit.Rg(6), Icx0=Windinit.Icx0(6), Icy0=Windinit.Icy0(6), C_w=Windinit.C_w(6), Vdc0=Windinit.Vdc0(6)}
      mask prompts: pitch "pitch_gain，pitch_max，pitch_rate"; Srotors "Start Rotor Speed"; Ex0 "Ex"; Ey0 "Ey"
      mask init:
      | pitch_gain=pitch(1);
      | pitch_max=pitch(2);
      | pitch_rate=pitch(3);
      | 
      | %该风机模型的基准容量
      | 
      | SwgeqB=SwgBi.*NN;
      mask DialogControl Container4 Prompt: PLL/Wind turbine
      mask DialogControl Container31 Prompt: Base value
      mask DialogControl Container23 Prompt: PLL
      mask DialogControl Container6 Prompt: inital value
      mask DialogControl Container5 Prompt: PI parameter
      mask DialogControl Container24 Prompt: Wind turbine
      mask DialogControl Container25 Prompt: pitch control
      mask DialogControl Container7 Prompt: Machine parameter
      mask DialogControl Container8 Prompt: Rotor
      mask DialogControl Container9 Prompt: Machine
      mask DialogControl Container10 Prompt: parameter
      mask DialogControl Container11 Prompt: inital value
      mask DialogControl Container12 Prompt: Rotor side control
      mask DialogControl Container13 Prompt: Control parameter
      mask DialogControl Container14 Prompt: Initial value
      mask DialogControl Container15 Prompt: reactive power
      mask DialogControl Container16 Prompt: Grid side control
      mask DialogControl Container17 Prompt: parameter
      mask DialogControl Container18 Prompt: reference
      mask DialogControl Container19 Prompt: inital value
      mask DialogControl Container20 Prompt: converter function
      mask DialogControl Container21 Prompt: inital value
      mask DialogControl Container22 Prompt: DC function
  Wind Generator - DFIG7 : Subsystem  mask{NN=Windinit.NN(7), SwgBi=Windinit.SwgBi(7), SmecBi=100, SgridB=SgridB, Atheta=Windinit.Atheta(7), Kppll=Windinit.Kppll_wind(7), Kipll=Windinit.Kipll_wind(7), pitch=[500 45 2], Srotors=1.3, H=Windinit.H(7), Wr0=Windinit.Wr0(7), Xa=Windinit.Xa(7), Xa1=Windinit.Xa1(7), Lm=Windinit.Lm(7), Lr=Windinit.Lr(7), Rs=Windinit.Rs(7), Ls=Windinit.Ls(7), Ta0=Windinit.Ta0(7), NPf=Windinit.NPf(7), Za=Windinit.Za{7}, Ex0=Windinit.Ex_ref(7), Ey0=Windinit.Ey_ref(7), wB=wB, KpP_rw=Windinit.KpP_rw(7), KiP_rw=Windinit.KiP_rw(7), KpId_rw=Windinit.KpId_rw(7), KiId_rw=Windinit.KiId_rw(7), KpQ_rw=Windinit.KpQ_rw(7), KiQ_rw=Windinit.KiQ_rw(7), KpIq_rw=Windinit.KpIq_rw(7), KiIq_rw=Windinit.KiIq_rw(7), Ird_ref=Windinit.Ird_ref(7), Irq_ref=Windinit.Irq_ref(7), Qs0=Windinit.Qs0(7), KpDC_gw=Windinit.KpDC_gw(7), KiDC_gw=Windinit.KiDC_gw(7), KpId_gw=Windinit.KpId_gw(7), KiId_gw=Windinit.KiId_gw(7), KpIq_gw=Windinit.KpIq_gw(7), KiIq_gw=Windinit.KiIq_gw(7), Vdc_w=Windinit.Vdc_w(7), Icd_ref=Windinit.Icd_ref(7), Icq_ref=Windinit.Icq_ref(7), Vcd_ref=Windinit.Vcd_ref(7), Vcq_ref=Windinit.Vcq_ref(7), Lg=Windinit.Lg(7), Rg=Windinit.Rg(7), Icx0=Windinit.Icx0(7), Icy0=Windinit.Icy0(7), C_w=Windinit.C_w(7), Vdc0=Windinit.Vdc0(7)}
      mask prompts: pitch "pitch_gain，pitch_max，pitch_rate"; Srotors "Start Rotor Speed"; Ex0 "Ex"; Ey0 "Ey"
      mask init:
      | pitch_gain=pitch(1);
      | pitch_max=pitch(2);
      | pitch_rate=pitch(3);
      | 
      | %该风机模型的基准容量
      | 
      | SwgeqB=SwgBi.*NN;
      mask DialogControl Container4 Prompt: PLL/Wind turbine
      mask DialogControl Container31 Prompt: Base value
      mask DialogControl Container23 Prompt: PLL
      mask DialogControl Container6 Prompt: inital value
      mask DialogControl Container5 Prompt: PI parameter
      mask DialogControl Container24 Prompt: Wind turbine
      mask DialogControl Container25 Prompt: pitch control
      mask DialogControl Container7 Prompt: Machine parameter
      mask DialogControl Container8 Prompt: Rotor
      mask DialogControl Container9 Prompt: Machine
      mask DialogControl Container10 Prompt: parameter
      mask DialogControl Container11 Prompt: inital value
      mask DialogControl Container12 Prompt: Rotor side control
      mask DialogControl Container13 Prompt: Control parameter
      mask DialogControl Container14 Prompt: Initial value
      mask DialogControl Container15 Prompt: reactive power
      mask DialogControl Container16 Prompt: Grid side control
      mask DialogControl Container17 Prompt: parameter
      mask DialogControl Container18 Prompt: reference
      mask DialogControl Container19 Prompt: inital value
      mask DialogControl Container20 Prompt: converter function
      mask DialogControl Container21 Prompt: inital value
      mask DialogControl Container22 Prompt: DC function
  Ixy : Outport
  tag scope: deltapes1=global, deltapes2=global, deltapes3=global
  wires:
  ES1/2(isxy) -> Mux4/1
  ES1/3(GBxy) -> Mux4/2
  ES3/2(isxy) -> Mux2/1
  ES3/3(GBxy) -> Mux2/2
  ES4/3(GBxy) -> Mux5/2
  ES5/2(isxy) -> Mux6/1
  ES5/3(GBxy) -> Mux6/2
  Mux4/1 -> Mux3/1
  Mux1/1 -> Mux3/2
  Demux1/1 -> ES1/1(us_xy)
  Demux1/2 -> ES2/1(us_xy)
  ES6/2(isxy) -> Mux10/1
  ES6/3(GBxy) -> Mux10/2
  ES7/2(isxy) -> Mux7/1
  ES7/3(GBxy) -> Mux7/2
  ES8/2(isxy) -> Mux8/1
  ES8/3(GBxy) -> Mux8/2
  Generator9/2(Igxy1) -> Mux11/1
  Generator9/3(GBxy) -> Mux11/2
  Generator10/2(Igxy1) -> Mux12/1
  Generator10/3(GBxy) -> Mux12/2
  Mux8/1 -> Mux9/3
  Mux11/1 -> Mux9/4
  Mux12/1 -> Mux9/5
  Demux2/3 -> ES8/1(us_xy)
  Demux2/4 -> Generator9/1(Vgxy)
  Demux2/5 -> Generator10/1(Vgxy)
  Mux13/1 -> Ixy/1
  Mux9/1 -> Mux13/2
  Mux3/1 -> Mux13/1
  Vxy/1 -> Demux/1
  Demux/1 -> Demux1/1
  Demux/2 -> Demux2/1
  Demux/3 -> [Vn], Scope10/1
  ES2/2(isxy) -> Mux1/1
  ES2/3(GBxy) -> Mux1/2
  ES4/2(isxy) -> Mux5/1
  ES1/1(m) -> [G1]
  ES2/1(m) -> [G2]
  ES3/1(m) -> Goto3/1
  ES4/1(m) -> Goto4/1
  ES5/1(m) -> Goto5/1
  ES6/1(m) -> Goto6/1
  ES7/1(m) -> Goto7/1
  ES8/1(m) -> [G8]
  Generator9/1(m) -> [G9]
  Generator10/1(m) -> [G10]
  [G1] -> Bus Selector/1
  Bus Selector/1 -> Scope/1  "<w>"
  [G8] -> Bus Selector27/1
  [G1] -> Bus Selector20/1
  [G2] -> Bus Selector21/1
  [G7] -> Bus Selector26/1
  [G10] -> Bus Selector29/1
  [G9] -> Bus Selector28/1
  [G4] -> Bus Selector23/1
  [G3] -> Bus Selector22/1
  [G6] -> Bus Selector25/1
  [G5] -> Bus Selector24/1
  Bus Selector20/1 -> Scope2/1  "<Pe>"
  Bus Selector21/1 -> Scope2/2  "<Pe>"
  Bus Selector22/1 -> Scope2/3  "<Pe>"
  Bus Selector23/1 -> Scope2/4  "<Pe>"
  Bus Selector24/1 -> Scope2/5  "<Pe>"
  Bus Selector25/1 -> Scope2/6  "<Pe>"
  Bus Selector28/1 -> Scope3/1  "<Pe>"
  Bus Selector29/1 -> Scope3/2  "<Pe>"
  [G2] -> Bus Selector1/1
  Bus Selector1/1 -> Scope/2  "<w>"
  [G3] -> Bus Selector2/1
  Bus Selector2/1 -> Scope/3  "<w>"
  [G4] -> Bus Selector3/1
  Bus Selector3/1 -> Scope/4  "<w>"
  [G5] -> Bus Selector4/1
  Bus Selector4/1 -> Scope/5  "<w>"
  [G6] -> Bus Selector5/1
  Bus Selector5/1 -> Scope/6  "<w>"
  [G10] -> Bus Selector9/1
  Bus Selector9/1 -> Scope1/2  "<f>"
  [G9] -> Bus Selector6/1
  Bus Selector6/1 -> Scope1/1  "<f>"
  From10/1 -> Gain17/1
  Mux24/1 -> Scope16/1  "Sim2Python"
  Gain17/1 -> Scope5/1, Mux24/3
  Mux14/1 -> Mux24/1
  Gain/1 -> Mux24/2, Scope4/1
  Bus Selector19/1 -> Mux14/6  "<Pe>"
  From19/1 -> Bus Selector19/1
  Bus Selector17/1 -> Mux14/4  "<Pe>"
  Bus Selector18/1 -> Mux14/5  "<Pe>"
  From15/1 -> Bus Selector15/1
  Bus Selector15/1 -> Mux14/2  "<Pe>"
  Bus Selector14/1 -> Mux14/1  "<Pe>"
  From17/1 -> Bus Selector17/1
  From18/1 -> Bus Selector18/1
  Bus Selector16/1 -> Mux14/3  "<Pe>"
  From14/1 -> Bus Selector14/1
  From16/1 -> Bus Selector16/1
  From82/1 -> Bus Selector10/1
  From83/1 -> Bus Selector11/1
  Bus Selector10/1 -> Mux14/7  "<Pe>"
  Bus Selector11/1 -> Mux14/8  "<Pe>"
  W_ES/1(W_ES) -> Goto11/1
  From12/1 -> Gain/1
  ROCOF_ES/1(ROCOF_ES) -> Goto12/1
  From11/1 -> Sum/1
  Sum3/1 -> Sum4/1
  From33/1 -> Sum1/2
  Sum/1 -> Sum3/1
  From42/1 -> Sum2/2
  From43/1 -> Sum5/1
  From30/1 -> Sum7/1
  Sum1/1 -> Sum3/2
  Sum7/1 -> Sum9/2
  From47/1 -> Sum6/2
  From46/1 -> Sum6/1
  Sum8/1 -> Sum9/1
  Sum2/1 -> Sum4/2
  Sum5/1 -> Sum8/1
  From13/1 -> Sum/2
  From44/1 -> Sum5/2
  From32/1 -> Sum1/1
  From34/1 -> Sum2/1
  From31/1 -> Sum7/2
  Sum6/1 -> Sum8/2
  From48/1 -> Sum10/1
  Sum10/1 -> Sum11/2
  From49/1 -> Sum10/2
  Sum11/1 -> Gain1/1
  Sum4/1 -> Sum11/1
  Gain1/1 -> Gain3/1
  Sum9/1 -> Sum12/1
  Sum12/1 -> Gain2/1
  From51/1 -> Sum13/2
  From50/1 -> Sum13/1
  Sum13/1 -> Sum12/2
  Gain2/1 -> Gain4/1
  Gain3/1 -> Goto13/1
  Gain4/1 -> Goto14/1
  From35/1 -> Scope6/1, Mux24/4
  From36/1 -> Scope7/1, Mux24/5
  [G7] -> Bus Selector7/1
  Bus Selector7/1 -> Scope/7  "<w>"
  [G8] -> Bus Selector8/1
  Bus Selector8/1 -> Scope/8  "<w>"
  Bus Selector26/1 -> Scope2/7  "<Pe>"
  Bus Selector27/1 -> Scope2/8  "<Pe>"
  Mux15/1 -> Gain19/1
  Add2/1 -> Gain18/1  "Pess1"
  From39/1 -> Mux15/1  "W1"
  Integrator/1 -> Scope8/1  "L2norm"
  Gain18/1 -> Add/2
  Add/1 -> Product/2, Math Function/1
  Product/1 -> Integrator/1
  Gain19/1 -> Add/1, Add2/1
  Math Function/1 -> Product/1
  From37/1 -> Mux15/2  "W2"
  From38/1 -> Mux15/4  "W4"
  From40/1 -> Mux15/3  "W3"
  From41/1 -> Mux15/5  "W5"
  From45/1 -> Mux15/6  "W6"
  From52/1 -> Mux15/7  "W7"
  From53/1 -> Mux15/8  "W8"
  Wind Generator - DFIG3/3(GBxy) -> Mux16/2
  Constant3/1 -> Wind Generator - DFIG3/1(Wind speed)
  Wind Generator - DFIG3/2(Igxy1) -> Mux16/1
  Wind Generator - DFIG3/1(m) -> [G3]
  Wind Generator - DFIG4/3(GBxy) -> Mux17/2
  Constant6/1 -> Wind Generator - DFIG4/1(Wind speed)
  Wind Generator - DFIG4/1(m) -> [G4]
  Wind Generator - DFIG4/2(Igxy1) -> Mux17/1
  Demux1/3 -> Wind Generator - DFIG3/2(Vsxy)
  Mux16/1 -> Mux3/3
  Demux1/4 -> Wind Generator - DFIG4/2(Vsxy)
  Mux17/1 -> Mux3/4
  Wind Generator - DFIG5/2(Igxy1) -> Mux18/1
  Wind Generator - DFIG6/1(m) -> [G6]
  Wind Generator - DFIG5/3(GBxy) -> Mux18/2
  Wind Generator - DFIG5/1(m) -> [G5]
  Wind Generator - DFIG6/2(Igxy1) -> Mux19/1
  Wind Generator - DFIG6/3(GBxy) -> Mux19/2
  Mux18/1 -> Mux3/5
  Constant4/1 -> Wind Generator - DFIG5/1(Wind speed)
  Demux1/5 -> Wind Generator - DFIG5/2(Vsxy)
  Mux19/1 -> Mux9/1
  Demux2/1 -> Wind Generator - DFIG6/2(Vsxy)
  Constant5/1 -> Wind Generator - DFIG6/1(Wind speed)
  Wind Generator - DFIG7/1(m) -> [G7]
  Constant1/1 -> Wind Generator - DFIG7/1(Wind speed)
  Demux2/2 -> Wind Generator - DFIG7/2(Vsxy)
  Wind Generator - DFIG7/2(Igxy1) -> Mux20/1
  Wind Generator - DFIG7/3(GBxy) -> Mux20/2
  Mux20/1 -> Mux9/2
  [P_list] -> Demux4/1
  Demux4/1 -> Sum16/1
  [fes2] -> Sum23/1
  Constant8/1 -> Sum20/2
  Python2Sim/1 -> Scope15/1, Demux5/1
  [fes2] -> Sum15/1
  Demux5/3 -> [deltapes3]
  [fg1] -> Sum19/1
  Demux5/1 -> [deltapes1]
  Demux5/2 -> [deltapes2]
  Constant2/1 -> Sum19/2
  Mux21/1 -> Scope13/1  "Sim2Python"
  Constant15/1 -> Sum15/2
  [fes1] -> Sum14/1
  Constant20/1 -> Sum23/2
  [fw5] -> Sum20/1
  Demux4/2 -> Sum16/2
  Constant7/1 -> Sum14/2
  Constant10/1 -> Sum24/2
  [G8] -> Bus Selector35/1
  Bus Selector35/1 -> Gain12/1  "<w>"
  [G2] -> Bus Selector13/1
  Bus Selector33/1 -> Gain10/1  "<w>"
  Gain7/1 -> [fw1], Scope9/3
  Gain6/1 -> [fes2], Scope9/2
  [G9] -> Bus Selector36/1
  [G7] -> Bus Selector34/1
  Gain11/1 -> [fw5], Scope9/7
  [G6] -> Bus Selector33/1
  Gain9/1 -> [fw3], Scope9/5
  Gain13/1 -> [fg1], Scope9/9
  Gain10/1 -> [fw4], Scope9/6
  Bus Selector37/1 -> Gain14/1  "<f>"
  Bus Selector12/1 -> Gain5/1  "<w>"
  Gain12/1 -> [fes3], Scope9/8
  Gain14/1 -> [fg2], Scope9/10
  Gain5/1 -> [fes1], Scope9/1
  [G5] -> Bus Selector32/1
  [G1] -> Bus Selector12/1
  Bus Selector30/1 -> Gain7/1  "<w>"
  [G3] -> Bus Selector30/1
  Bus Selector31/1 -> Gain8/1  "<w>"
  Bus Selector34/1 -> Gain11/1  "<w>"
  [G10] -> Bus Selector37/1
  [G4] -> Bus Selector31/1
  Bus Selector32/1 -> Gain9/1  "<w>"
  Gain8/1 -> [fw2], Scope9/4
  Bus Selector13/1 -> Gain6/1  "<w>"
  Bus Selector36/1 -> Gain13/1  "<f>"
  Sum19/1 -> Mux21/1
  Sum14/1 -> Mux21/2
  Sum20/1 -> Mux21/3
  Constant9/1 -> Sum21/2
  [fg2] -> Sum21/1
  Sum21/1 -> Mux21/4
  Sum23/1 -> Mux21/5
  Sum24/1 -> Mux21/6
  [fw1] -> Sum24/1
  Sum15/1 -> Mux21/7
  [fw3] -> Add1/2
  [fw2] -> Add1/1
  Constant18/1 -> Divide1/2
  Add1/1 -> Divide1/1
  [fw4] -> Add1/3
  Divide1/1 -> Sum22/1
  Constant11/1 -> Sum22/2
  Sum22/1 -> Mux21/8
  Sum16/1 -> Mux21/9
  Demux4/3 -> Mux21/10
  Demux4/4 -> Mux21/11
  Demux/4 -> [P_list]
  Demux3/1 -> Scope11/1
  [P_list] -> Demux3/1
  Demux3/3 -> Scope14/1
  Demux3/2 -> Scope12/1
  Demux3/4 -> Scope17/1
  Clock/1 -> Mux21/12
